simulink model "Fig422"  (R2014b)
settings: Solver=ode3  StartTime=0.0  StopTime=5.24288  FixedStep=2e-5  RelTol=1e-3
libraries: commrandsrc2 x1
settings Model: Creator=Dennis Silage  LastModifiedBy=Silage
settings DataIOCC: SignalLoggingSaveFormat=ModelDataLogs
settings OptimizationCC: ExpressionDepthLimit=2147483647  InitFltsAndDblsToZero=on
settings DebuggingCC: UnderspecifiedInitializationDetection=Classic  MergeDetectMultiDrivingBlocksExec=none  FcnCallInpInsideContextMsg=UseLocalSettings  StateNameClashWarn=warning
settings GRTTargetCC: CombineOutputUpdateFcns=off  GRTInterface=on

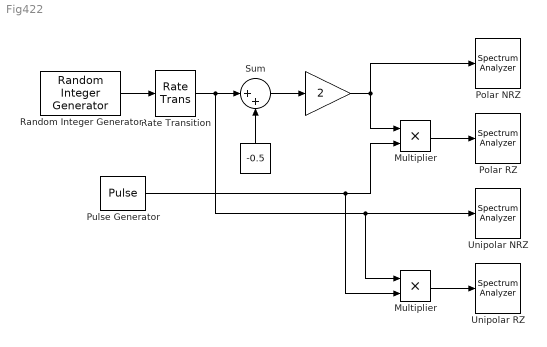
== system Fig422 ==
  " " : Constant  Value=-0.5
  "   " : Gain  Gain=2
  " Rate Transition" : RateTransition  OutPortSampleTime=2e-5
  Multiplier : Product  RndMeth=Zero
  "Multiplier " : Product  RndMeth=Zero
  Polar NRZ : SpectrumAnalyzer
  Polar RZ : SpectrumAnalyzer
  Pulse Generator : DiscretePulseGenerator  Period=50  PulseWidth=25  SampleTime=2e-5
  Random Integer Generator : commrandsrc2/Random Integer Generator  mul=2  seed=randseed  Ts=1e-3  frameBased=off  sampPerFrame=1  orient=off  outDataType=double
  Sum : Sum  Inputs=|++
  Unipolar NRZ : SpectrumAnalyzer
  Unipolar RZ : SpectrumAnalyzer
  wires:
  Sum/1 -> "   "/1
  " "/1 -> Sum/2
  "   "/1 -> "Multiplier "/1, Polar NRZ/1
  Pulse Generator/1 -> "Multiplier "/2, Multiplier/2
  "Multiplier "/1 -> Polar RZ/1
  Multiplier/1 -> Unipolar RZ/1
  Random Integer Generator/1 -> " Rate Transition"/1
  " Rate Transition"/1 -> Sum/1, Multiplier/1, Unipolar NRZ/1
